simulink subsystem "UserInputsMotorSwapHost"  (R2024b)
settings: Solver=VariableStepAuto  StartTime=0.0  StopTime=10.0  RelTol=1e-3
values from neighbouring files (symbols this model uses):
  Ts = T_pwm    [mcbMotorSwapData.m]
  Ts_serialIn = 50e-3    (= 0.05)    [MicrochipTargetMotorControlData.m]
libraries: simulink x1, svdutilitieslib x1
settings Model: Creator=The MathWorks, Inc.  LastModifiedBy=snarayan
settings RTWCC: GPUComputeCapability=3.5

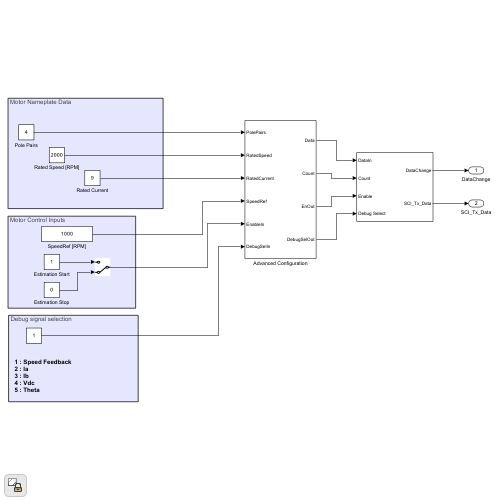
[thumbnail: Simulink's stored preview of the top-level diagram]
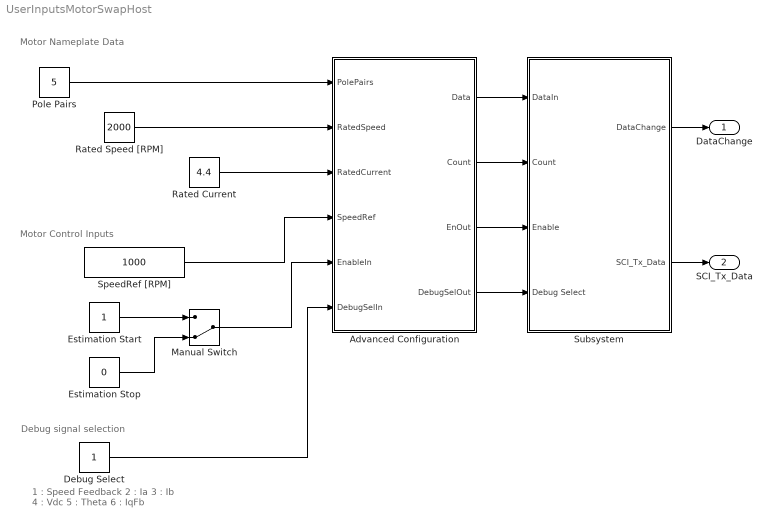
== system UserInputsMotorSwapHost ==
  note: Motor Control Inputs
  note: Debug signal selection
  note: 1 : Speed Feedback
      | 2 : Ia
      | 3 : Ib
      | 4 : Vdc
      | 5 : Theta
      | 6 : IqFb
  note: Motor Nameplate Data
  Advanced Configuration : Subsystem
  Debug Select : Constant  OutDataTypeStr=uint8  SampleTime=-1
  Estimation Start : Constant  OutDataTypeStr=uint16  SampleTime=-1
  Estimation Stop : Constant  Value=0  OutDataTypeStr=uint16  SampleTime=-1
  Manual Switch : ManualSwitch  CurrentSetting=0
  Pole Pairs : Constant  Value=5  OutDataTypeStr=single
  Rated Current : Constant  Value=4.4  OutDataTypeStr=single
  Rated Speed [RPM] : Constant  Value=2000  OutDataTypeStr=single
  SpeedRef [RPM] : Constant  Value=1000  OutDataTypeStr=single  SampleTime=-1
  Subsystem : Subsystem
  DataChange : Outport
  SCI_Tx_Data : Outport  Port=2
  wires:
  Subsystem/1(DataChange) -> DataChange/1
  Subsystem/2(SCI_Tx_Data) -> SCI_Tx_Data/1
  Estimation Stop/1 -> Manual Switch/2
  Estimation Start/1 -> Manual Switch/1
  Manual Switch/1 -> Advanced Configuration/5(EnableIn)
  Pole Pairs/1 -> Advanced Configuration/1(PolePairs)
  Rated Current/1 -> Advanced Configuration/3(RatedCurrent)
  Rated Speed [RPM]/1 -> Advanced Configuration/2(RatedSpeed)
  SpeedRef [RPM]/1 -> Advanced Configuration/4(SpeedRef)
  Advanced Configuration/2(Count) -> Subsystem/2(Count)
  Advanced Configuration/1(Data) -> Subsystem/1(DataIn)
  Advanced Configuration/3(EnOut) -> Subsystem/3(Enable)
  Debug Select/1 -> Advanced Configuration/6(DebugSelIn)
  Advanced Configuration/4(DebugSelOut) -> Subsystem/4(Debug Select)

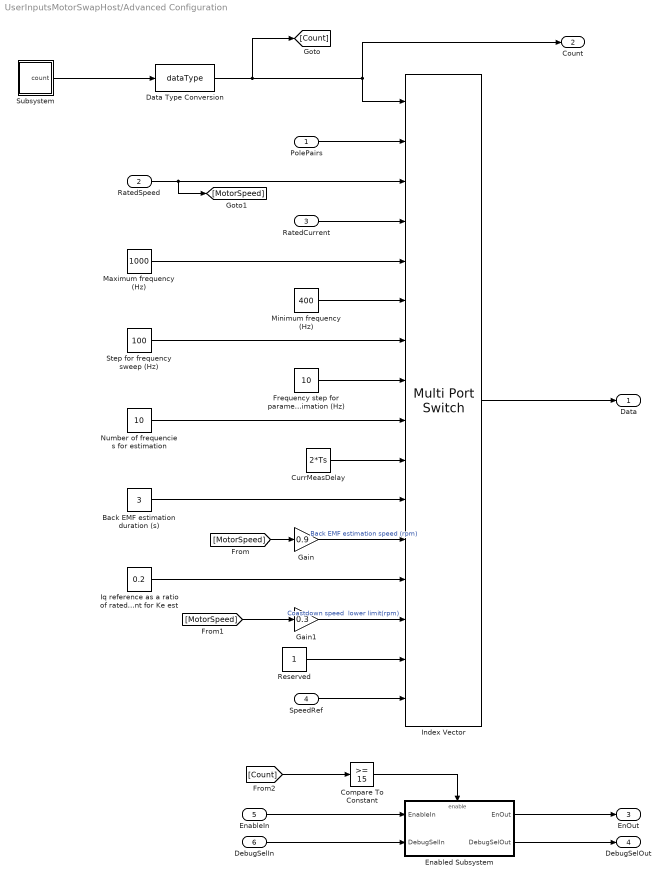
== system UserInputsMotorSwapHost/Advanced Configuration ==
  PolePairs : Inport
  RatedSpeed : Inport  Port=2
  RatedCurrent : Inport  Port=3
  SpeedRef : Inport  Port=4
  EnableIn : Inport  Port=5
  DebugSelIn : Inport  Port=6
  " Maximum frequency (Hz)" : Constant  Value=1000  OutDataTypeStr=dataType
  Back EMF estimation duration (s) : Constant  Value=3  OutDataTypeStr=dataType
  Compare To Constant : simulink/Logic and Bit Operations/Compare To Constant  relop=>=  const=15  OutDataTypeStr=boolean
  CurrMeasDelay : Constant  Value=2*Ts  OutDataTypeStr=dataType
  Data Type Conversion : DataTypeConversion  OutDataTypeStr=dataType  RndMeth=Simplest  SaturateOnIntegerOverflow=off
  Enabled Subsystem : Subsystem  TreatAsAtomicUnit=on
  Frequency step for parameter estimation (Hz) : Constant  Value=10  OutDataTypeStr=dataType
  Gain : Gain  Gain=0.9  RndMeth=Simplest  OutDataTypeStr=Inherit: Same as input
  Gain1 : Gain  Gain=0.3  RndMeth=Simplest  OutDataTypeStr=Inherit: Same as input
  Index Vector : MultiPortSwitch  Inputs=15  OutDataTypeStr=dataType  RndMeth=Simplest  SaturateOnIntegerOverflow=off  InputSameDT=off
  Iq reference as a ratio of rated motor current for Ke est : Constant  Value=0.2  OutDataTypeStr=dataType
  Minimum frequency (Hz) : Constant  Value=400  OutDataTypeStr=dataType
  Number of frequencies for estimation : Constant  Value=10  OutDataTypeStr=dataType
  Reserved : Constant  OutDataTypeStr=single
  Step for frequency sweep (Hz) : Constant  Value=100  OutDataTypeStr=dataType
  Subsystem : Subsystem  mask(Counter){upperLimit=15, sampleTime=Ts_serialIn * 10}
      mask prompts: upperLimit "Upper Limit"; sampleTime "Sample Time"
      mask help: Conter starts from 1 and reaches Upper Limit using given sample time in steps of 1.
  Data : Outport
  Count : Outport  Port=2
  EnOut : Outport  Port=3
  DebugSelOut : Outport  Port=4
  wires:
  Reserved/1 -> Index Vector/15
  " Maximum frequency (Hz)"/1 -> Index Vector/5
  Minimum frequency (Hz)/1 -> Index Vector/6
  Step for frequency sweep (Hz)/1 -> Index Vector/7
  Frequency step for parameter estimation (Hz)/1 -> Index Vector/8
  Number of frequencies for estimation/1 -> Index Vector/9
  CurrMeasDelay/1 -> Index Vector/10
  Back EMF estimation duration (s)/1 -> Index Vector/11
  Gain/1 -> Index Vector/12  "Back EMF estimation speed (rpm)"
  Iq reference as a ratio of rated motor current for Ke est/1 -> Index Vector/13
  Gain1/1 -> Index Vector/14  "Coastdown speed  lower limit(rpm)"
  SpeedRef/1 -> Index Vector/16
  Compare To Constant/1 -> Enabled Subsystem/Enable
  [Count] -> Compare To Constant/1
  Enabled Subsystem/2(DebugSelOut) -> DebugSelOut/1
  DebugSelIn/1 -> Enabled Subsystem/2(DebugSelIn)
  Enabled Subsystem/1(EnOut) -> EnOut/1
  EnableIn/1 -> Enabled Subsystem/1(EnableIn)
  [MotorSpeed] -> Gain1/1
  [MotorSpeed] -> Gain/1
  RatedCurrent/1 -> Index Vector/4
  PolePairs/1 -> Index Vector/2
  RatedSpeed/1 -> Index Vector/3, [MotorSpeed]
  Data Type Conversion/1 -> Index Vector/1, Count/1, [Count]
  Index Vector/1 -> Data/1
  Subsystem/1(count) -> Data Type Conversion/1

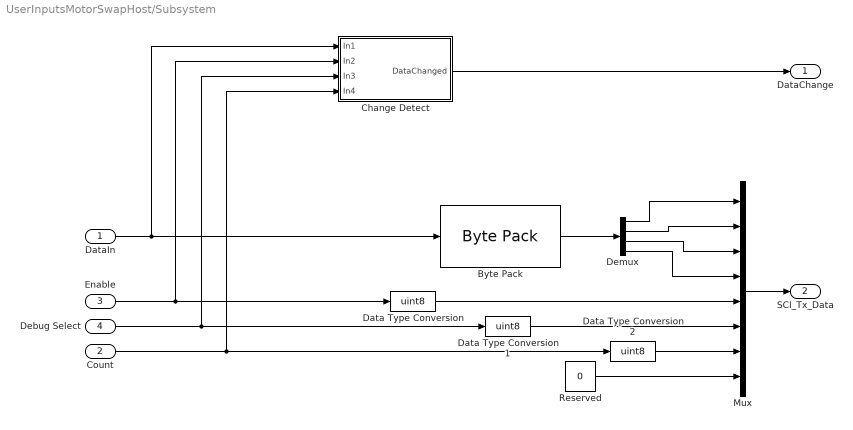
== system UserInputsMotorSwapHost/Subsystem ==
  DataIn : Inport
  Count : Inport  Port=2
  Enable : Inport  Port=3
  Debug Select : Inport  Port=4
  Byte Pack : svdutilitieslib/Byte Pack  maskPackedDataType=uint8  datatypes={'single'}  byteAlign=1  blockPlatform=tic2000
  Change Detect : Subsystem
  Data Type Conversion : DataTypeConversion  OutDataTypeStr=uint8  RndMeth=Simplest  SaturateOnIntegerOverflow=off
  Data Type Conversion1 : DataTypeConversion  OutDataTypeStr=uint8  RndMeth=Simplest  SaturateOnIntegerOverflow=off
  Data Type Conversion2 : DataTypeConversion  OutDataTypeStr=uint8  RndMeth=Simplest  SaturateOnIntegerOverflow=off
  Demux : Demux
  Mux : Mux  Inputs=8
  Reserved : Constant  Value=0  OutDataTypeStr=uint8
  DataChange : Outport
  SCI_Tx_Data : Outport  Port=2
  wires:
  Byte Pack/1 -> Demux/1
  Reserved/1 -> Mux/8
  Data Type Conversion2/1 -> Mux/7
  Data Type Conversion1/1 -> Mux/6
  Data Type Conversion/1 -> Mux/5
  Demux/1 -> Mux/1
  Demux/4 -> Mux/4
  Demux/2 -> Mux/2
  Demux/3 -> Mux/3
  Count/1 -> Data Type Conversion2/1, Change Detect/4(In4)
  DataIn/1 -> Byte Pack/1, Change Detect/1(In1)
  Change Detect/1(DataChanged) -> DataChange/1
  Mux/1 -> SCI_Tx_Data/1
  Enable/1 -> Data Type Conversion/1, Change Detect/2(In2)
  Debug Select/1 -> Data Type Conversion1/1, Change Detect/3(In3)

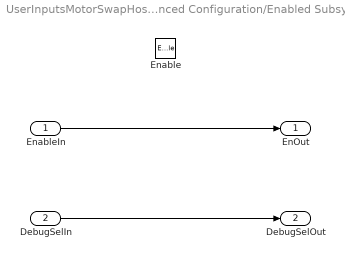
== system UserInputsMotorSwapHost/Advanced Configuration/Enabled Subsystem ==
  EnableIn : Inport
  DebugSelIn : Inport  Port=2
  Enable : EnablePort
  EnOut : Outport
  DebugSelOut : Outport  Port=2
  wires:
  DebugSelIn/1 -> DebugSelOut/1
  EnableIn/1 -> EnOut/1

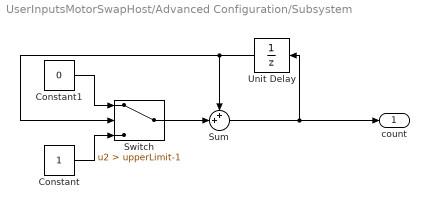
== system UserInputsMotorSwapHost/Advanced Configuration/Subsystem ==
  Constant : Constant  OutDataTypeStr=uint8  SampleTime=sampleTime
  Constant1 : Constant  Value=0  OutDataTypeStr=uint8  SampleTime=sampleTime
  Sum : Sum  Inputs=++|  OutDataTypeStr=uint8  AccumDataTypeStr=uint8  RndMeth=Simplest
  Switch : Switch  Criteria=u2 > Threshold  Threshold=upperLimit-1  OutDataTypeStr=uint8  RndMeth=Simplest  SaturateOnIntegerOverflow=off  InputSameDT=off
  Unit Delay : UnitDelay  SampleTime=-1  HasFrameUpgradeWarning=on
  count : Outport
  wires:
  Constant/1 -> Switch/3
  Switch/1 -> Sum/2
  Unit Delay/1 -> Sum/1, Switch/2
  Sum/1 -> Unit Delay/1, count/1
  Constant1/1 -> Switch/1

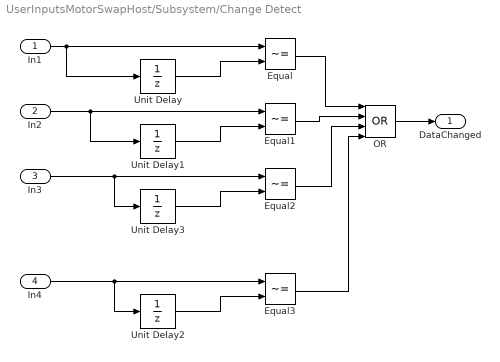
== system UserInputsMotorSwapHost/Subsystem/Change Detect ==
  In1 : Inport
  In2 : Inport  Port=2
  In3 : Inport  Port=3
  In4 : Inport  Port=4
  Equal{,1..3} (4 alike) : RelationalOperator  Operator=~=  OutDataTypeStr=boolean  RndMeth=Simplest  InputSameDT=off
  OR : Logic  Operator=OR  Inputs=4  IconShape=distinctive  AllPortsSameDT=off  OutDataTypeStr=boolean
  Unit Delay{,1..3} (4 alike) : UnitDelay  SampleTime=-1  HasFrameUpgradeWarning=on
  DataChanged : Outport
  wires:
  Equal3/1 -> OR/4
  In4/1 -> Unit Delay2/1, Equal3/1
  Unit Delay2/1 -> Equal3/2
  Unit Delay3/1 -> Equal2/2
  Unit Delay1/1 -> Equal1/2
  In1/1 -> Equal/1, Unit Delay/1
  In2/1 -> Equal1/1, Unit Delay1/1
  Equal/1 -> OR/1
  Unit Delay/1 -> Equal/2
  Equal1/1 -> OR/2
  In3/1 -> Equal2/1, Unit Delay3/1
  OR/1 -> DataChanged/1
  Equal2/1 -> OR/3
